simulink model "vagolap"  (Simulink 8.1)
settings: Solver=ode45  StartTime=0.0  StopTime=10.0  RelTol=1e-3
values from neighbouring files (symbols this model uses):
  sample = 10e-5    (= 0.0001)    [Symmetry_ini_COPY.m]    (also in animated_norms.m; save_data.m)
settings Model: Creator=Neukirchner László  LastModifiedBy=Neukirchner László
settings DataIOCC: SignalLoggingSaveFormat=Dataset
settings OptimizationCC: ExpressionDepthLimit=128
settings DebuggingCC: FcnCallInpInsideContextMsg=EnableAllAsError
settings GRTTargetCC: CombineOutputUpdateFcns=on  GRTInterface=off

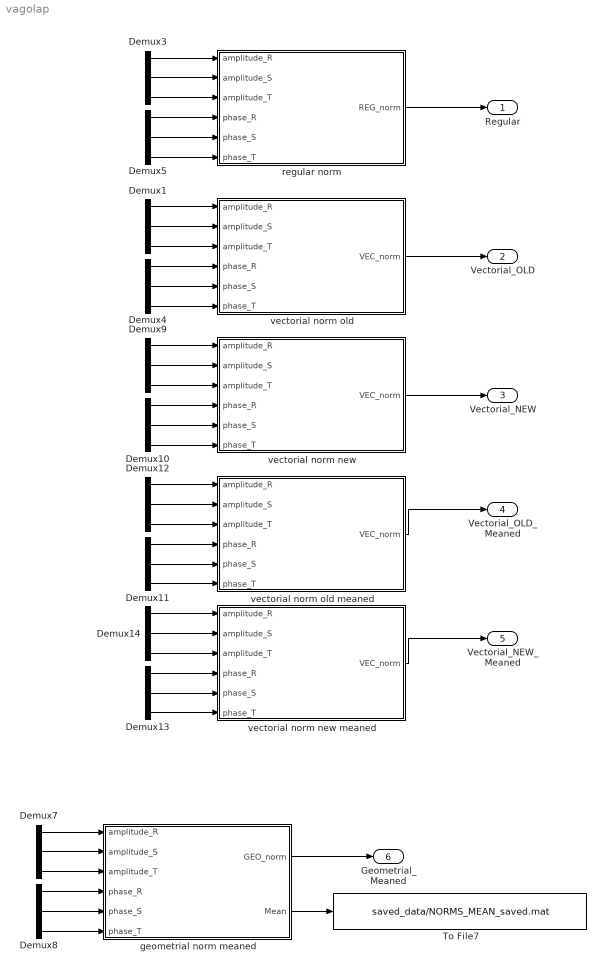
== system vagolap ==
  Demux{1,3..5,7..14} (12 alike) : Demux  Outputs=3
  To File7 : ToFile  Filename=saved_data/NORMS_MEAN_saved.mat  MatrixName=NORMS_MEAN_saved  SaveFormat=Timeseries  SampleTime=sample
  geometrial norm meaned : MATLAB Function  TreatAsAtomicUnit=on
  regular norm : MATLAB Function  TreatAsAtomicUnit=on
  vectorial norm new : MATLAB Function  TreatAsAtomicUnit=on
  vectorial norm new meaned : MATLAB Function  TreatAsAtomicUnit=on
  vectorial norm old : MATLAB Function  TreatAsAtomicUnit=on
  vectorial norm old meaned : MATLAB Function  TreatAsAtomicUnit=on
  Regular : Outport
  Vectorial_OLD : Outport  Port=2
  Vectorial_NEW : Outport  Port=3
  Vectorial_OLD_Meaned : Outport  Port=4
  Vectorial_NEW_Meaned : Outport  Port=5
  Geometrial_Meaned : Outport  Port=6
  wires:
  Demux1/1 -> vectorial norm old/1(amplitude_R)
  Demux1/2 -> vectorial norm old/2(amplitude_S)
  Demux1/3 -> vectorial norm old/3(amplitude_T)
  Demux4/1 -> vectorial norm old/4(phase_R)
  Demux4/2 -> vectorial norm old/5(phase_S)
  Demux4/3 -> vectorial norm old/6(phase_T)
  vectorial norm old/1(VEC_norm) -> Vectorial_OLD/1
  regular norm/1(REG_norm) -> Regular/1
  Demux3/1 -> regular norm/1(amplitude_R)
  Demux3/2 -> regular norm/2(amplitude_S)
  Demux3/3 -> regular norm/3(amplitude_T)
  Demux5/1 -> regular norm/4(phase_R)
  Demux5/2 -> regular norm/5(phase_S)
  Demux5/3 -> regular norm/6(phase_T)
  Demux9/1 -> vectorial norm new/1(amplitude_R)
  Demux9/2 -> vectorial norm new/2(amplitude_S)
  Demux9/3 -> vectorial norm new/3(amplitude_T)
  Demux10/1 -> vectorial norm new/4(phase_R)
  Demux10/2 -> vectorial norm new/5(phase_S)
  Demux10/3 -> vectorial norm new/6(phase_T)
  vectorial norm new/1(VEC_norm) -> Vectorial_NEW/1
  ? -> Demux5/1
  ? -> Demux4/1
  ? -> Demux11/1
  ? -> Demux10/1
  Demux12/1 -> vectorial norm old meaned/1(amplitude_R)
  Demux12/2 -> vectorial norm old meaned/2(amplitude_S)
  Demux12/3 -> vectorial norm old meaned/3(amplitude_T)
  Demux11/1 -> vectorial norm old meaned/4(phase_R)
  Demux11/2 -> vectorial norm old meaned/5(phase_S)
  Demux11/3 -> vectorial norm old meaned/6(phase_T)
  vectorial norm old meaned/1(VEC_norm) -> Vectorial_OLD_Meaned/1
  ? -> Demux3/1
  ? -> Demux1/1
  ? -> Demux12/1
  ? -> Demux13/1
  ? -> Demux14/1
  ? -> Demux9/1
  Demux14/1 -> vectorial norm new meaned/1(amplitude_R)
  Demux14/2 -> vectorial norm new meaned/2(amplitude_S)
  Demux14/3 -> vectorial norm new meaned/3(amplitude_T)
  Demux13/1 -> vectorial norm new meaned/4(phase_R)
  Demux13/2 -> vectorial norm new meaned/5(phase_S)
  Demux13/3 -> vectorial norm new meaned/6(phase_T)
  vectorial norm new meaned/1(VEC_norm) -> Vectorial_NEW_Meaned/1
  Demux7/1 -> geometrial norm meaned/1(amplitude_R)
  Demux7/2 -> geometrial norm meaned/2(amplitude_S)
  Demux7/3 -> geometrial norm meaned/3(amplitude_T)
  Demux8/1 -> geometrial norm meaned/4(phase_R)
  Demux8/2 -> geometrial norm meaned/5(phase_S)
  Demux8/3 -> geometrial norm meaned/6(phase_T)
  geometrial norm meaned/1(GEO_norm) -> Geometrial_Meaned/1
  ? -> Demux8/1
  ? -> Demux7/1
  geometrial norm meaned/2(Mean) -> To File7/1

== matlab function vectorial norm old ==
  data: amplitude_R input double; VEC_norm output double; amplitude_S input double; amplitude_T input double; phase_R input double; phase_S input double; phase_T input double
function VEC_norm = fcn(amplitude_R,amplitude_S,amplitude_T,phase_R,phase_S,phase_T)
%#codegen

  
   N=complex(0);
   V_real=complex([0,0,0]');
  %V_012=complex([0,0,0]');
   V_real(1)=amplitude_R.*exp(1i*phase_R);
   V_real(2)=amplitude_S.*exp(1i*phase_S);
   V_real(3)=amplitude_T.*exp(1i*phase_T); 

   R_error=230*exp(1j*-0/360*2*pi)  -V_real(1);
   S_error=230*exp(1j*-120/360*2*pi)-V_real(2);
   T_error=230*exp(1j*-240/360*2*pi)-V_real(3);
   %VEC_norm=abs(R_error*S_error)+abs(R_error*T_error)+abs(S_error*T_error);
   N=R_error*S_error+R_error*T_error+S_error*T_error;
   VEC_norm=abs(N);

== matlab function regular norm ==
  data: amplitude_R input double; REG_norm output double; amplitude_S input double; amplitude_T input double; phase_R input double; phase_S input double; phase_T input double
function REG_norm = fcn(amplitude_R,amplitude_S,amplitude_T,phase_R,phase_S,phase_T)
%#codegen

 A=(1/3)*[1,                1,                  1;...
          1,      exp(1i*120/360*2*pi),        exp(1i*240/360*2*pi);...
          1,      exp(1i*240/360*2*pi),       exp(1i*120/360*2*pi)];
   
   V_real=complex([0,0,0]');
   V_012=complex([0,0,0]');
   V_real(1)=amplitude_R.*exp(1i*phase_R);
   V_real(2)=amplitude_S.*exp(1i*phase_S);
   V_real(3)=amplitude_T.*exp(1i*phase_T); 
   V_012=A*V_real;
   REG_norm=(abs(V_012(3))/abs(V_012(2)))*100;

== matlab function geometrial norm meaned ==
  data: amplitude_R input double; GEO_norm output double; amplitude_S input double; amplitude_T input double; phase_R input double; phase_S input double; phase_T input double; Mean output double
function [GEO_norm,Mean] = fcn(amplitude_R,amplitude_S,amplitude_T,phase_R,phase_S,phase_T)
%#codegen

x1=[0,0,0,0];
y1=[0,0,0,0];
x2=[0,0,0,0];
y2=[0,0,0,0];

GEO_norm=0;
Mean=0;

coder.extrinsic('geometry_solver')

        %% Ideal parameters
        Mean=(amplitude_R+amplitude_S+amplitude_T)/3;
        Amplitude_1=[Mean,Mean,Mean];                     %[V]
        %Phase_1=[-1.5855,2.6033,0.5089];
        Phase_1=[0,-2/3*pi,-4/3*pi];                     %[rad]
      
        %% Real parameters
        Amplitude_2=[amplitude_R,amplitude_S,amplitude_T];
        Phase_2=[phase_R,phase_S,phase_T];
        %Extension of the vectors with the first element to get closed triangles on
        %plots and for use as polygons
        Amplitude_1_ex=[Amplitude_1 Amplitude_1(1)];
        Phase_1_ex=[Phase_1 Phase_1(1)];
        Amplitude_2_ex=[Amplitude_2 Amplitude_2(1)];
        Phase_2_ex=[Phase_2 Phase_2(1)];
        
        GEO_norm=geometry_solver(Amplitude_1_ex, Phase_1_ex, Amplitude_2_ex, Phase_2_ex);

== matlab function vectorial norm new ==
  data: amplitude_R input double; VEC_norm output double; amplitude_S input double; amplitude_T input double; phase_R input double; phase_S input double; phase_T input double
function VEC_norm = fcn(amplitude_R,amplitude_S,amplitude_T,phase_R,phase_S,phase_T)
%#codegen

  
   N=complex(0);
   V_real=complex([0,0,0]');
  %V_012=complex([0,0,0]');
   V_real(1)=amplitude_R.*exp(1i*phase_R);
   V_real(2)=amplitude_S.*exp(1i*phase_S);
   V_real(3)=amplitude_T.*exp(1i*phase_T); 

   R_error=230*exp(1j*-0/360*2*pi)  -V_real(1);
   S_error=230*exp(1j*-120/360*2*pi)-V_real(2);
   T_error=230*exp(1j*-240/360*2*pi)-V_real(3);
   VEC_norm=abs(R_error*S_error)+abs(R_error*T_error)+abs(S_error*T_error);
   %N=R_error*S_error+R_error*T_error+S_error*T_error;
   %VEC_norm=abs(N);

== matlab function vectorial norm old meaned ==
  data: amplitude_R input double; VEC_norm output double; amplitude_S input double; amplitude_T input double; phase_R input double; phase_S input double; phase_T input double
function VEC_norm  = fcn(amplitude_R,amplitude_S,amplitude_T,phase_R,phase_S,phase_T)
%#codegen

   Mean=0;
   Mean=(amplitude_R+amplitude_S+amplitude_T)/3;
   N=complex(0);
   V_real=complex([0,0,0]');
  %V_012=complex([0,0,0]');
   V_real(1)=Mean.*exp(1i*phase_R);
   V_real(2)=Mean.*exp(1i*phase_S);
   V_real(3)=Mean.*exp(1i*phase_T); 

   R_error=230*exp(1j*-0/360*2*pi)  -V_real(1);
   S_error=230*exp(1j*-120/360*2*pi)-V_real(2);
   T_error=230*exp(1j*-240/360*2*pi)-V_real(3);
   %VEC_norm=abs(R_error*S_error)+abs(R_error*T_error)+abs(S_error*T_error);
   N=R_error*S_error+R_error*T_error+S_error*T_error;
   VEC_norm=abs(N);

== matlab function vectorial norm new meaned ==
  data: amplitude_R input double; VEC_norm output double; amplitude_S input double; amplitude_T input double; phase_R input double; phase_S input double; phase_T input double
function VEC_norm  = fcn(amplitude_R,amplitude_S,amplitude_T,phase_R,phase_S,phase_T)
%#codegen

  
   Mean=0;
   Mean=(amplitude_R+amplitude_S+amplitude_T)/3;
   N=complex(0);
   V_real=complex([0,0,0]');
  %V_012=complex([0,0,0]');
   V_real(1)=Mean.*exp(1i*phase_R);
   V_real(2)=Mean.*exp(1i*phase_S);
   V_real(3)=Mean.*exp(1i*phase_T);  

   R_error=230*exp(1j*-0/360*2*pi)  -V_real(1);
   S_error=230*exp(1j*-120/360*2*pi)-V_real(2);
   T_error=230*exp(1j*-240/360*2*pi)-V_real(3);
   VEC_norm=abs(R_error*S_error)+abs(R_error*T_error)+abs(S_error*T_error);
   %N=R_error*S_error+R_error*T_error+S_error*T_error;
   %VEC_norm=abs(N);
